simulink model "SecondOrderMultibitSC"  (R2023b)
settings: Solver=VariableStepDiscrete  StartTime=0.0  StopTime=(N-1)*ts  RelTol=1e-3  EnableMultiTasking=on
undefined symbols (not defined in the file): Adc, Ain, cs1a, fin, gm, io, ts, Vn, vosp, Vr
libraries: fesclib x2, quantidlib x1
settings Model: SimulationMode=accelerator  Creator=jrosa  LastModifiedBy=pablo
settings SolverCC: AlgebraicLoopSolver=TrustRegion
settings DataIOCC: LimitDataPoints=on  SaveFormat=Array  ReturnWorkspaceOutputs=off
settings OptimizationCC: ReuseModelBlockBuffer=off  ExpressionDepthLimit=2147483647  InitFltsAndDblsToZero=on  LifeSpan=inf
settings DebuggingCC: SaveWithParameterizedLinksMsg=none  UnderspecifiedInitializationDetection=Classic  MergeDetectMultiDrivingBlocksExec=none  SignalResolutionControl=TryResolveAllWithWarning  SolverPrmCheckMsg=warning  MultiTaskDSMMsg=warning  MultiTaskCondExecSysMsg=none  FcnCallInpInsideContextMsg=warning  UnconnectedInputMsg=warning  UnconnectedOutputMsg=warning  UnconnectedLineMsg=warning  StateNameClashWarn=warning  SFUnexpectedBacktrackingDiag=warning  SFNoUnconditionalDefaultTransitionDiag=warning  SFExecutionAtInitializationDiag=none  ArithmeticOperatorsInVariantConditions=warning
settings HardwareCC: ProdBitPerPointer=32  ProdBitPerSizeT=32  ProdBitPerPtrDiffT=32  ProdLargestAtomicFloat=None  ProdIntDivRoundTo=Undefined  ProdEndianess=Unspecified  ProdWordSize=32  ProdHWDeviceType=32-bit Generic
settings ModelReferenceCC: PropagateSignalLabelsOutOfModel=off
settings SFSimCC: SimUseLocalCustomCode=off  CustomCodeUndefinedFunction=UseInterfaceOnly
settings RTWCC: RTWUseLocalCustomCode=off
settings CodeAppCC: StateflowObjectComments=on
settings GRTTargetCC: TargetFcnLib=ansi_tfl_tmw.mat  TargetLangStandard=C89/C90 (ANSI)  CombineOutputUpdateFcns=off  GRTInterface=on
settings ConfigComp: CovMetricSettings=dw  CovSaveCumulativeToWorkspaceVar=on  CovSaveSingleToWorkspaceVar=on  CovExternalEMLEnable=off

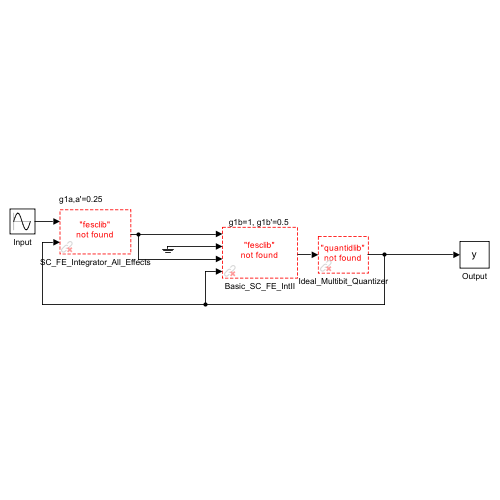
[thumbnail: Simulink's stored preview of the top-level diagram]
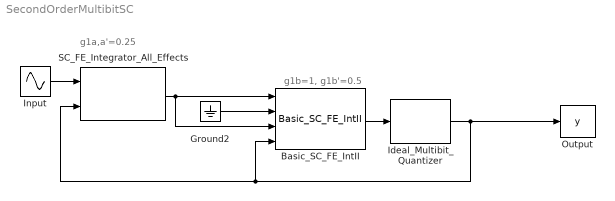
== system SecondOrderMultibitSC ==
  note: g1a,a'=0.25
  note: g1b=1, g1b'=0.5
  Basic_SC_FE_IntII : fesclib/Basic_SC_FE_IntII  opspos=vosp  opsneg=-vosp  c2=ci1b  c11=cs1b  c12=cs1b  phi=phi1  ts=ts
  Ground2 : Ground
  Ideal_Multibit_Quantizer : quantidlib/Ideal_Multibit_Quantizer  Vhigh=vhigh  Vlow=vlow  n_bits=B  Xfs=2*Vr  phi=phi1  ts=ts  qid=cuant
  Input : Sin  Amplitude=Ain  Frequency=2*pi*fin  SampleTime=0
  Output : ToWorkspace  VariableName=y  SampleTime=ts
  SC_FE_Integrator_All_Effects : fesclib/SC_FE_Integrator_All_Effects  c=[cs1a,4*cs1a,0,0]  var=[0,Vn,275,300]  ops=[vosp,-vosp]  ao=[Adc,gm,io]  avnl=[0,0,0,0]  cp=[0.05e-12,0.05e-12,2.5e-12]  phi=phi1  ts=ts  settlingon=on  setin=off  idown=int1  idnext=int1
      link override Capacidades: Value=1e-11
      link override From: GotoTag=int1
      link override Goto: GotoTag=int1
  wires:
  Basic_SC_FE_IntII/1 -> Ideal_Multibit_Quantizer/1
  Ground2/1 -> Basic_SC_FE_IntII/2
  SC_FE_Integrator_All_Effects/1 -> Basic_SC_FE_IntII/1, Basic_SC_FE_IntII/3
  Input/1 -> SC_FE_Integrator_All_Effects/1
  Ideal_Multibit_Quantizer/1 -> Basic_SC_FE_IntII/4, SC_FE_Integrator_All_Effects/2, Output/1
